simulink model "TuneBaseDriver"  (R2020b)
settings: Solver=VariableStepAuto  StartTime=0.0  StopTime=100  RelTol=1e-3
undefined symbols (not defined in the file): DiscIntNeverNeededParam, maxAngles, ts_camera
libraries: simulink_extras x1
settings Model: DataDictionary=Dictionary.sldd  EnableAccessToBaseWorkspace=off  Creator=alons  LastModifiedBy=elbit

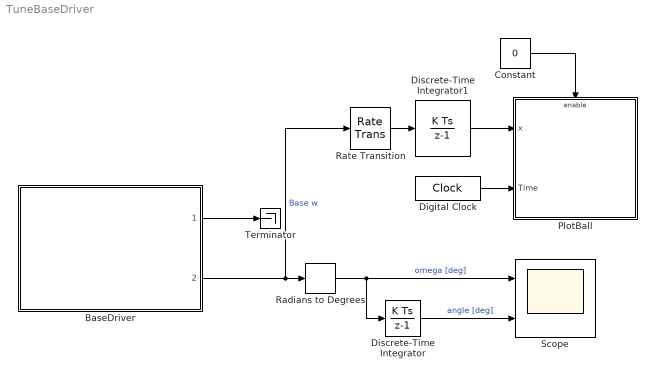
== system TuneBaseDriver ==
  BaseDriver : Subsystem  ReferencedSubsystem=BaseDriver
  Constant : Constant  Value=0  SampleTime=0.016
      settings: OpenFcn=|
      | if get_param(gcbh,'value')-48
      |    set_param(gcbh,'value','0','backgroundcolor','red');
      | else
      |    set_param(gcbh,'value','1','backgroundcolor','green');
      | end
  Digital Clock : DigitalClock  SampleTime=ts_camera
  Discrete-Time Integrator : DiscreteIntegrator  SampleTime=-1  ICPrevOutput=DiscIntNeverNeededParam  ICPrevScaledInput=DiscIntNeverNeededParam
  Discrete-Time Integrator1 : DiscreteIntegrator  SampleTime=-1  ICPrevOutput=DiscIntNeverNeededParam  ICPrevScaledInput=DiscIntNeverNeededParam
  PlotBall : Subsystem
      settings: OpenFcn=|
      | UserData = get_param([gcb,'/AnimationSfcn'],'UserData');
      | Fig = UserData.Figure;
      | if ishghandle(Fig,'figure');
      |    %bring to the front:
      |    figure(Fig);
      | end
      mask Display:
      | t=linspace(0,2*pi,20);
      | plot(cos(t),sin(t));
      | 
      | x=[-0.4,-0.4,0.6,-0.4];
      | y=[-0.5,0.5,0,-0.5];
      | plot(x,y)
      | 
      | color('black');
      | disp('Plot Ball');
  Radians to Degrees : simulink_extras/Transformations/Radians to Degrees
  Rate Transition : RateTransition
  Scope : Scope  NumInputPorts=2
  Terminator : Terminator
  wires:
  BaseDriver/1 -> Terminator/1
  BaseDriver/2 -> Rate Transition/1, Radians to Degrees/1  "Base w"
  Discrete-Time Integrator/1 -> Scope/2  "angle [deg]"
  Radians to Degrees/1 -> Discrete-Time Integrator/1, Scope/1  "omega [deg]"
  Rate Transition/1 -> Discrete-Time Integrator1/1
  Constant/1 -> PlotBall/Enable
  Discrete-Time Integrator1/1 -> PlotBall/1(x)
  Digital Clock/1 -> PlotBall/2(Time)

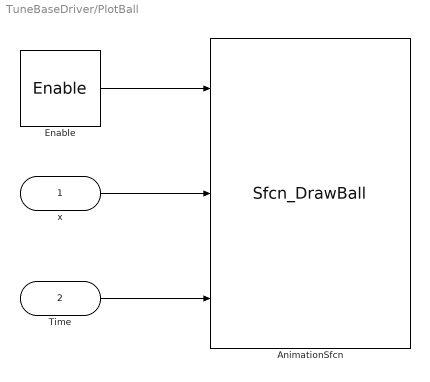
== system TuneBaseDriver/PlotBall ==
  x : Inport
  Time : Inport  Port=2
  Enable : EnablePort  StatesWhenEnabling=reset  ShowOutputPort=on
  AnimationSfcn : M-S-Function  FunctionName=Sfcn_DrawBall  Parameters=[maxAngles(1)*[-2,2];maxAngles(2)*[-2,2];maxAngles(3)*[-2,2]]
  wires:
  x/1 -> AnimationSfcn/2
  Enable/1 -> AnimationSfcn/1
  Time/1 -> AnimationSfcn/3
